simulink model "mpc_control_casadi_c_implement3"  (R2023a)
settings: Solver=VariableStepAuto  StartTime=0.0  StopTime=20  RelTol=1e-3
undefined symbols (not defined in the file or in its folder): k, v
libraries: Solver_SF x1, vehdynlibsteering x1, slpidlib x1
settings Model: Creator=Miakho  LastModifiedBy=15003
settings OptimizationCC: ReuseModelBlockBuffer=off

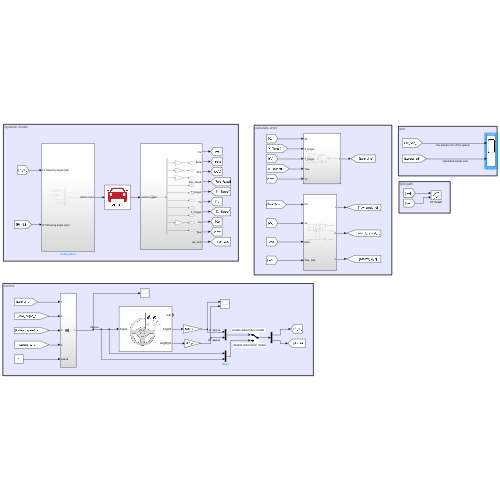
[thumbnail: Simulink's stored preview of the top-level diagram]
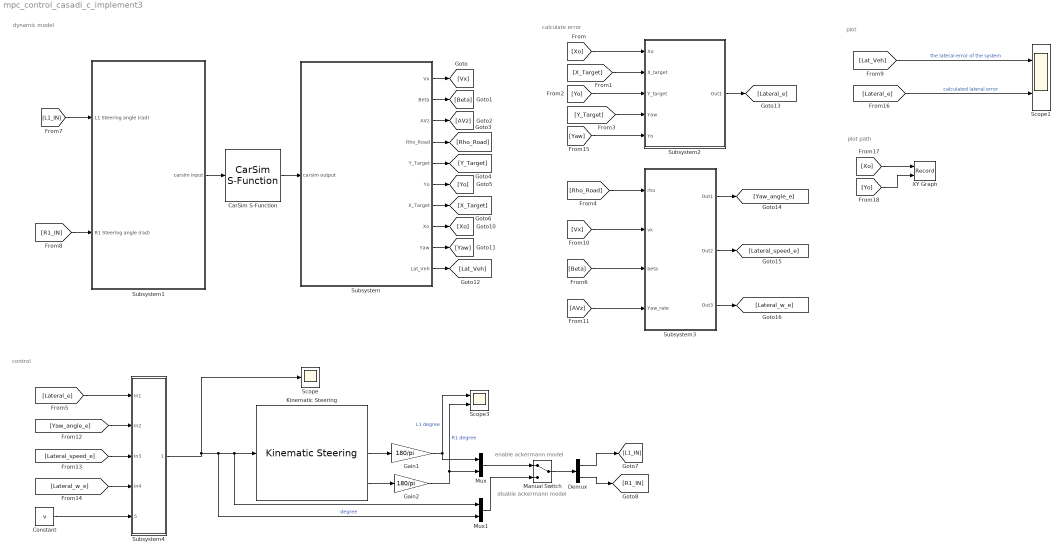
== system mpc_control_casadi_c_implement3 ==
  note: disable ackermann model
  note: enable ackermann model
  note: plot
  note: plot path
  note: control
  note: calculate error
  note: dynamic model
  CarSim S-Function : Solver_SF/CarSim S-Function  Priority=1  SIMFILE=simfile.sim  Run_RTs=off  vs_state_ind=Run  StopMode_ind=Vehicle Model
  Constant : Constant  Value=v
  Demux : Demux  Outputs=2
  Gain1 : Gain  Gain=180/pi
  Gain2 : Gain  Gain=180/pi
  Kinematic Steering : vehdynlibsteering/Kinematic Steering  StrgType=Ackerman  StrgRatioType=Constant  Loc=Front  NrmlFctr=1  TrckWdth=1.575  WhlBase=2.950  Db=0  StrgRng=1.25*pi  StrgAngBpts="[-6.2832   -5.0265   -3.7699   -2.5133   -1.2566         0    1.2566    2.5133    3.7699    5.0265    6.2832]"  StrgRatioTbl=|  StrgRatio=100  PctAckIn=off  PctAck=100  PctAckTbl=ones(1,11)*100  StrgArmLngth=0.1  RckCsLngth=0.5  TieRodLngth=0.248  D=0.2  PnnRadius=0.00085818  PnnRadiusTbl="[0.0055    0.0055    0.0056    0.0057    0.0058    0.0057    0.0057    0.0057    0.0056    0.0055    0.0055]"  RodLngth=0.1  ParaArmLngth=0.9  aMode=2
      | [13.5000   13.3750   13.2500   13.1250   13.0000   13.0000   13.0000   13.1250   13.2500   13.3750   13.5000
      | ]
  Manual Switch : ManualSwitch
  Mux : Mux  Inputs=2
  Mux1 : Mux  Inputs=2
  Scope : Scope
  Scope1 : Scope  NumInputPorts=2
  Scope3 : Scope  NumInputPorts=2
  Subsystem : Subsystem
  Subsystem1 : Subsystem
  Subsystem2 : Subsystem
  Subsystem3 : Subsystem
  Subsystem4 : Subsystem
  XY Graph : Record  FileSettingsInternal="{\"entries\":[{\"content\":{\"excelSettings\":{\"content\":{},\"type\":\"Streamout.ExcelSettings\"}},\"type\":\"Streamout.FileSettingStorage\",\"uuid\":\"\"}],\"packageUris\":[\"http:\\/\\/schema.mathworks.com\\/mf0\\/streamout_blocks\\/R2020a\"],\"version\":\"1.0\"}"  Layout=[1 1]  SignalsInternal="{\"entries\":[{\"content\":{\"signals\":[{\"content\":{\"blockPath\":[],\"dimensions\":[1],\"domain\":\"\",\"lineColor\":\"#a2142f\",\"plots\":[1],\"port\":1,\"sid\":[\"\"],\"signalID\":21157,\"signalName\":\"From17\"},\"type\":\"RecordBlkView.Signal\",\"uuid\":\"\"},{\"content\":{\"blockPath\":[],\"dimensions\":[1],\"domain\":\"\",\"lineColor\":\"#139fff\",\"plots\":[1],\"port\":2,\"sid\":[\"\"],\"signalID\":21161,\"signalName\":\"From18\"},\"type\":\"RecordBlkView.Signal\",\"uuid\":\"\"}]},\"type\":\"RecordBlkView.InputSignals\",\"uuid\":\"\"}],\"packageUris\":[\"http:\\/\\/schema.mathworks.com\\/mf0\\/streamout_blocks\\/R2020a\"],\"version\":\"1.0\"}"  VisualizationBindings="{\"xyplotplugin\":{\"info\":[{\"series\":[{\"bindingParametersList\":[{\"parameter\":\"X-Axis\",\"signalID\":21157,\"signalName\":\"From17\"},{\"parameter\":\"Y-Axis\",\"signalID\":21161,\"signalName\":\"From18\"}],\"seriesID\":28898}],\"subplotID\":1}]}}"  CompatibilityTag=XY
  wires:
  Kinematic Steering/2 -> Gain1/1
  Subsystem1/1(carsim input) -> CarSim S-Function/1
  Subsystem/10(Lat_Veh) -> [Lat_Veh]
  [R1_IN] -> Subsystem1/2(R1 Steering angle (rad))
  [Rho_Road] -> Subsystem3/1(rho)
  Subsystem4/1(Out1) -> Mux1/2, Mux1/1, Kinematic Steering/1, Scope/1  "degree"
  Gain1/1 -> Mux/1, Scope3/1  "L1 degree"
  Subsystem/1(Vx) -> [Vx]
  Subsystem/9(Yaw) -> [Yaw]
  [Y_Target] -> Subsystem2/4(Yaw)
  [Yaw] -> Subsystem2/5(Yo)
  Subsystem/6(Yo) -> [Yo]
  Gain2/1 -> Scope3/2, Mux/2  "R1 degree"
  [Xo] -> XY Graph/1
  [Lateral_e] -> Subsystem4/1(In1)
  Subsystem/4(Rho_Road) -> [Rho_Road]
  Subsystem/7(X_Target) -> [X_Target]
  Subsystem3/3(Out3) -> [Lateral_w_e]
  [Lateral_w_e] -> Subsystem4/4(In4)
  [Lateral_e] -> Scope1/2  "calculated lateral error"
  [Vx] -> Subsystem3/2(vx)
  [Lat_Veh] -> Scope1/1  "the lateral error of the system"
  Subsystem/2(Beta) -> [Beta]
  [X_Target] -> Subsystem2/2(X_target)
  [Yo] -> XY Graph/2
  Subsystem/3(AVz) -> [AVz]
  [L1_IN] -> Subsystem1/1(L1 Steering angle (rad))
  CarSim S-Function/1 -> Subsystem/1(carsim output)
  Subsystem3/1(Out1) -> [Yaw_angle_e]
  [Yo] -> Subsystem2/3(Y_target)
  [Lateral_speed_e] -> Subsystem4/3(In3)
  Subsystem/5(Y_Target) -> [Y_Target]
  [Beta] -> Subsystem3/3(beta)
  Subsystem2/1(Out1) -> [Lateral_e]
  Subsystem/8(Xo) -> [Xo]
  Kinematic Steering/3 -> Gain2/1
  Subsystem3/2(Out2) -> [Lateral_speed_e]
  [Yaw_angle_e] -> Subsystem4/2(In2)
  [Xo] -> Subsystem2/1(Xo)
  [AVz] -> Subsystem3/4(Yaw_rate)
  Mux/1 -> Manual Switch/1
  Mux1/1 -> Manual Switch/2
  Manual Switch/1 -> Demux/1
  Demux/1 -> [L1_IN]
  Demux/2 -> [R1_IN]
  Constant/1 -> Subsystem4/5(speed)

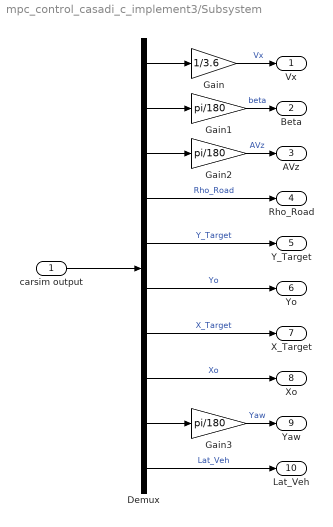
== system mpc_control_casadi_c_implement3/Subsystem ==
  carsim output : Inport
  Demux : Demux  Outputs=10
  Gain : Gain  Gain=1/3.6
  Gain1 : Gain  Gain=pi/180
  Gain2 : Gain  Gain=pi/180
  Gain3 : Gain  Gain=pi/180
  Vx : Outport
  Beta : Outport  Port=2
  AVz : Outport  Port=3
  Rho_Road : Outport  Port=4
  Y_Target : Outport  Port=5
  Yo : Outport  Port=6
  X_Target : Outport  Port=7
  Xo : Outport  Port=8
  Yaw : Outport  Port=9
  Lat_Veh : Outport  Port=10
  wires:
  Demux/3 -> Gain2/1
  Demux/1 -> Gain/1
  carsim output/1 -> Demux/1
  Demux/6 -> Yo/1  "Yo"
  Demux/7 -> X_Target/1  "X_Target"
  Demux/4 -> Rho_Road/1  "Rho_Road"
  Demux/2 -> Gain1/1
  Demux/5 -> Y_Target/1  "Y_Target"
  Demux/8 -> Xo/1  "Xo"
  Demux/9 -> Gain3/1
  Demux/10 -> Lat_Veh/1  "Lat_Veh"
  Gain/1 -> Vx/1  "Vx"
  Gain1/1 -> Beta/1  "beta"
  Gain2/1 -> AVz/1  "AVz"
  Gain3/1 -> Yaw/1  "Yaw"

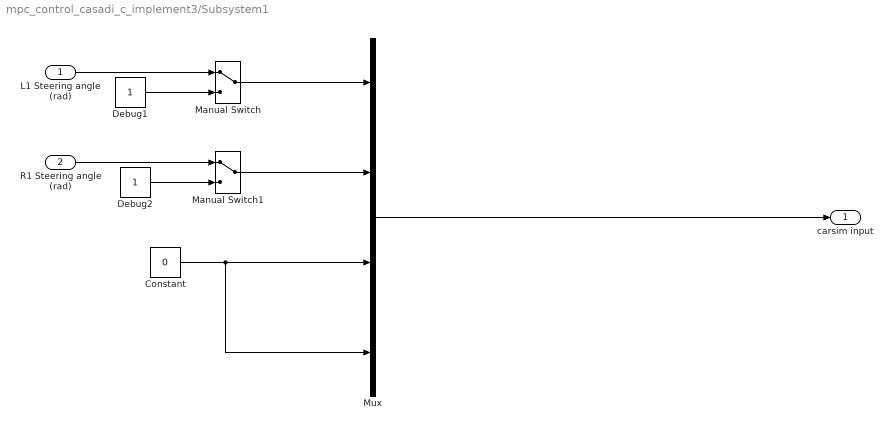
== system mpc_control_casadi_c_implement3/Subsystem1 ==
  L1 Steering angle (rad) : Inport
  R1 Steering angle (rad) : Inport  Port=2
  Constant : Constant  Value=0
  Debug1 : Constant
  Debug2 : Constant
  Manual Switch : ManualSwitch
  Manual Switch1 : ManualSwitch
  Mux : Mux
  carsim input : Outport
  wires:
  R1 Steering angle (rad)/1 -> Manual Switch1/1
  L1 Steering angle (rad)/1 -> Manual Switch/1
  Constant/1 -> Mux/4, Mux/3
  Debug1/1 -> Manual Switch/2
  Manual Switch/1 -> Mux/1
  Manual Switch1/1 -> Mux/2
  Debug2/1 -> Manual Switch1/2
  Mux/1 -> carsim input/1

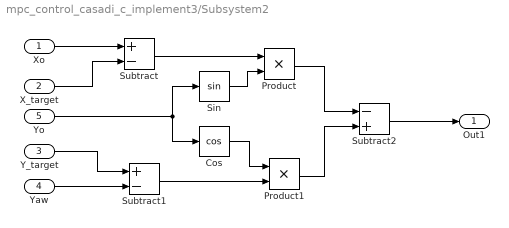
== system mpc_control_casadi_c_implement3/Subsystem2 ==
  Xo : Inport
  X_target : Inport  Port=2
  Y_target : Inport  Port=3
  Yaw : Inport  Port=4
  Yo : Inport  Port=5
  Cos : Trigonometry  Operator=cos
  Product : Product
  Product1 : Product
  Sin : Trigonometry
  Subtract : Sum  Inputs=+-
  Subtract1 : Sum  Inputs=+-
  Subtract2 : Sum  Inputs=-+
  Out1 : Outport
  wires:
  Y_target/1 -> Subtract1/1
  Subtract1/1 -> Product1/2
  Subtract/1 -> Product/1
  Product/1 -> Subtract2/1
  X_target/1 -> Subtract/2
  Sin/1 -> Product/2
  Yo/1 -> Sin/1, Cos/1
  Cos/1 -> Product1/1
  Product1/1 -> Subtract2/2
  Yaw/1 -> Subtract1/2
  Subtract2/1 -> Out1/1
  Xo/1 -> Subtract/1

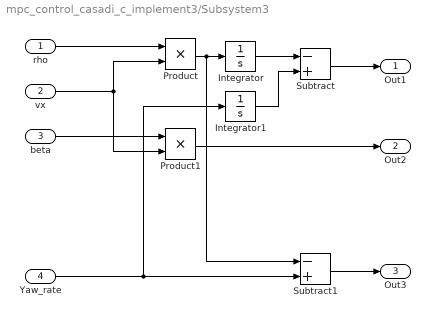
== system mpc_control_casadi_c_implement3/Subsystem3 ==
  rho : Inport
  vx : Inport  Port=2
  beta : Inport  Port=3
  Yaw_rate : Inport  Port=4
  Integrator : Integrator
  Integrator1 : Integrator
  Product : Product
  Product1 : Product
  Subtract : Sum  Inputs=-+
  Subtract1 : Sum  Inputs=-+
  Out1 : Outport
  Out2 : Outport  Port=2
  Out3 : Outport  Port=3
  wires:
  Integrator/1 -> Subtract/1
  Integrator1/1 -> Subtract/2
  vx/1 -> Product1/2, Product/2
  Yaw_rate/1 -> Subtract1/2, Integrator1/1
  Product/1 -> Subtract1/1, Integrator/1
  rho/1 -> Product/1
  Subtract/1 -> Out1/1
  Subtract1/1 -> Out3/1
  beta/1 -> Product1/1
  Product1/1 -> Out2/1

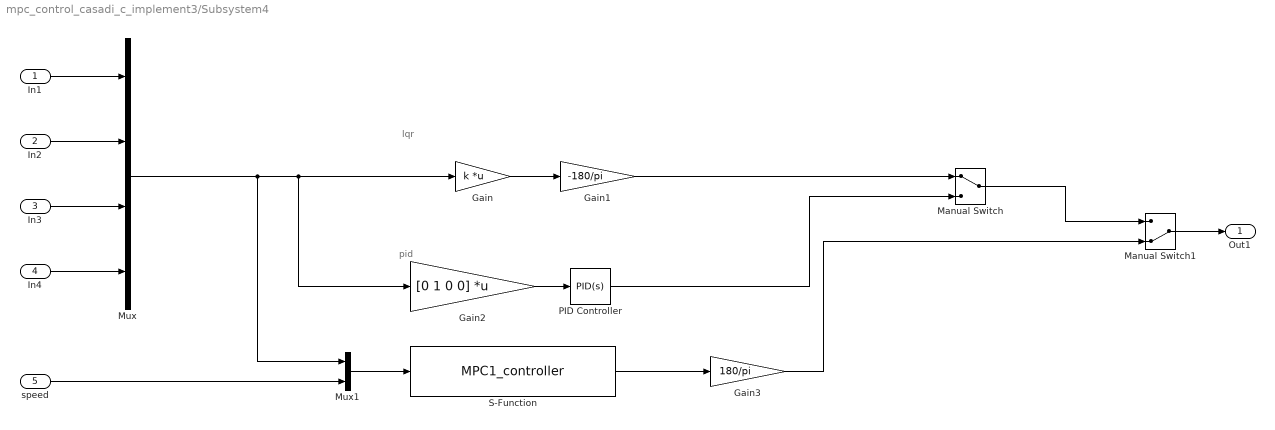
== system mpc_control_casadi_c_implement3/Subsystem4 ==
  note: pid
  note: lqr
  In1 : Inport
  In2 : Inport  Port=2
  In3 : Inport  Port=3
  In4 : Inport  Port=4
  speed : Inport  Port=5
  Gain : Gain  Gain=k  Multiplication=Matrix(K*u)
  Gain1 : Gain  Gain=-180/pi
  Gain2 : Gain  Gain=[0 1 0 0]  Multiplication=Matrix(K*u)
  Gain3 : Gain  Gain=180/pi
  Manual Switch : ManualSwitch
  Manual Switch1 : ManualSwitch  CurrentSetting=0
  Mux : Mux
  Mux1 : Mux  Inputs=2
  PID Controller : slpidlib/PID Controller  Controller=PID  Form=Parallel  TimeDomain=Continuous-time  UseExternalTs=off  SampleTime=-1  IntegratorMethod=Forward Euler  FilterMethod=Forward Euler  ControllerParametersSource=internal  P=-5  I=0  UseKiTs=off  D=-100  N=100  UseFilter=on  TunerSelectOption=Transfer Function Based (PID Tuner App)  InitialConditionSource=internal  InitialConditionForIntegrator=0  InitialConditionForFilter=0  DifferentiatorICPrevScaledInput=0  ExternalReset=none  TrackingMode=off  Kt=1  LimitOutput=off  SatLimitsSource=internal  UpperSaturationLimit=inf  LowerSaturationLimit=-inf  LinearizeAsGain=on  AntiWindupMode=none  Kb=1  LimitIntegrator=off  UpperIntegratorSaturationLimit=inf  LowerIntegratorSaturationLimit=-inf  POutMin=[]  POutMax=[]  IOutMin=[]  IOutMax=[]  DOutMin=[]  DOutMax=[]  NOutMin=[]  NOutMax=[]  SumOutMin=[]  SumOutMax=[]  SaturationOutMin=[]  SaturationOutMax=[]  PParamMin=[]  PParamMax=[]  IParamMin=[]  IParamMax=[]  DParamMin=[]  DParamMax=[]  NParamMin=[]  NParamMax=[]  KbParamMin=[]  KbParamMax=[]  KtParamMin=[]  KtParamMax=[]  KbOutMin=[]  KbOutMax=[]  KtOutMin=[]  KtOutMax=[]  IntegratorOutMin=[]  IntegratorOutMax=[]  FilterOutMin=[]  FilterOutMax=[]  SumI1OutMin=[]  SumI1OutMax=[]  SumI2OutMin=[]  SumI2OutMax=[]  SumI3OutMin=[]  SumI3OutMax=[]  SumI4OutMin=[]  SumI4OutMax=[]  SumDOutMin=[]  SumDOutMax=[]  DifferentiatorOutMin=[]  DifferentiatorOutMax=[]  FilterDiffOutCoefMin=[]  FilterDiffOutCoefMax=[]  ReciprocalOutMin=[]  ReciprocalOutMax=[]  SumDenOutMin=[]  SumDenOutMax=[]  SumNumOutMin=[]  SumNumOutMax=[]  DivideOutMin=[]  DivideOutMax=[]  UdiffTsProdOutMin=[]  UdiffTsProdOutMax=[]  NTsProdOutMin=[]  NTsProdOutMax=[]  UintegralTsProdOutMin=[]  UintegralTsProdOutMax=[]  UngainTsProdOutMin=[]  UngainTsProdOutMax=[]  ClampingZeroOutDataTypeStr=Inherit: Inherit via back propagation  ClampingZeroOutMin=[]  ClampingZeroOutMax=[]  FilterDenConstantOutDataTypeStr=Inherit: Inherit via back propagation  FilterDenConstantOutMin=[]  FilterDenConstantOutMax=[]  PCopyOutDataTypeStr=Inherit: Inherit via back propagation  PCopyOutMin=[]  PCopyOutMax=[]  NCopyOutDataTypeStr=Inherit: Inherit via back propagation  NCopyOutMin=[]  NCopyOutMax=[]  IntegratorContinuousStateAttributes=''  IntegratorStateMustResolveToSignalObject=off  IntegratorRTWStateStorageClass=Auto  FilterContinuousStateAttributes=''  FilterStateMustResolveToSignalObject=off  FilterRTWStateStorageClass=Auto  ParallelPVariant=InternalParameters  IdealPVariant=Disabled  IVariant=InternalParameters  DVariant=InternalParameters  IntegratorVariant=Continuous  SatVariant=Disabled  AWVariant=Passthrough  PCopyVariant=Disabled  TRVariant=Disabled  FdbkBlocksVariant=Forward  IdealPFdbkVariant=Disabled  SatFdbkVariant=Disabled  DerivativeFilterVariant=ContFilter  NVariant=InternalParameters  NCopyVariant=Disabled  FilterICVariant=InternalICsFilter  IntegratorICVariant=InternalICs  ExternalResetVariant=Disabled  TRSumVariant=Passthrough  SumFdbkVariant=Disabled  SumVariant=Sum_PID  TsampFilterVariant=InternalTs  TsampNgainVariant=Passthrough  TsampIntegralVariant=Disabled_SignalSpec  ExternalSaturationOutDataTypeStr=Inherit: Same as second input
  S-Function : S-Function  FunctionName=MPC1_controller  SFunctionDeploymentMode=off  EnableBusSupport=off
  Out1 : Outport
  wires:
  In4/1 -> Mux/4
  In2/1 -> Mux/2
  In1/1 -> Mux/1
  In3/1 -> Mux/3
  Gain/1 -> Gain1/1
  Gain1/1 -> Manual Switch/1
  Manual Switch/1 -> Manual Switch1/1
  Mux/1 -> Mux1/1, Gain2/1, Gain/1
  Gain2/1 -> PID Controller/1
  PID Controller/1 -> Manual Switch/2
  Mux1/1 -> S-Function/1
  speed/1 -> Mux1/2
  Manual Switch1/1 -> Out1/1
  S-Function/1 -> Gain3/1
  Gain3/1 -> Manual Switch1/2
